simulink model "RefModel_RigInput"  (R2015b)
settings: configuration reference "CenterOutReachConfigSet" (kept outside this file)
undefined symbols (not defined in the file or in its folder): DiscIntNeverNeededParam, handAccelerationX, handAccelerationY, handAccelerationZ, HandSource, SimulinkParameter_TunableRigConfig
libraries: simulink x11, libBusSerialize x7, slrtlib x2, dspindex x1, libIntelSMI x1, xpcnilib x1, dspswit3 x1, commfilt2 x1
settings Model: Creator=djoshea  LastModifiedBy=shenoylab
settings ConfigSetRef: SourceLocation=Base Workspace

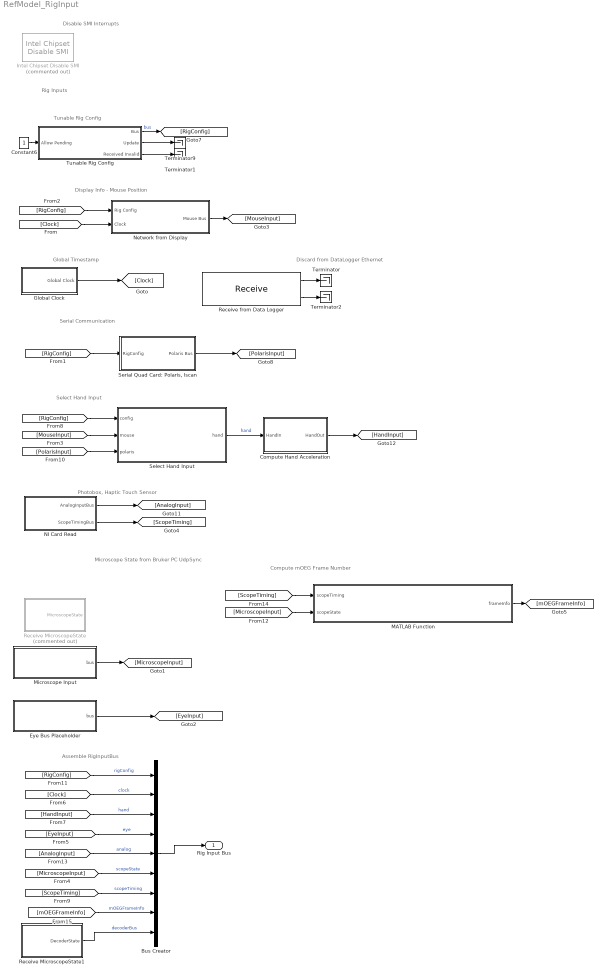
== system RefModel_RigInput ==
  note: Display Info - Mouse Position
  note: Serial Communication
  note: Global Timestamp
  note: Photobox, Haptic Touch Sensor
  note: Tunable Rig Config
  note: Select Hand Input
  note: Assemble RigInputBus
  note: Microscope State from Bruker PC UdpSync
  note: Disable SMI Interrupts
  note: Discard from DataLogger Ethernet
  note: Rig Inputs
  note: Compute mOEG Frame Number
  Bus Creator : BusCreator  Inputs=9  OutDataTypeStr=Bus: RigInputBus  NonVirtualBus=on
  Compute Hand Acceleration : Subsystem
  Constant6 : Constant  OutDataTypeStr=uint8
  Eye Bus Placeholder : MATLAB Function  AncestorBlock=libBusSerialize/Initialize Bus  TreatAsAtomicUnit=on  mask(Initialize Bus Block){busType=Bus: EyeInputBus}
      mask prompts: busType "Bus Type:"
      mask help: This block simply wraps an initializeBus_BusName() function and is useful for debugging where bus inputs are required. It acts essentially like a ground source for bus types.
      mask init:
      | BusSerialize.maskInitializeBusBlockUpdate(gcb);
  Global Clock : Subsystem
  Intel Chipset Disable SMI : libIntelSMI/Intel Chipset Disable SMI  Commented=on
  MATLAB Function : MATLAB Function  TreatAsAtomicUnit=on
  Microscope Input : MATLAB Function  AncestorBlock=libBusSerialize/Initialize Bus  TreatAsAtomicUnit=on  mask(Initialize Bus Block){busType=Bus: MicroscopeStateBus}
      mask prompts: busType "Bus Type:"
      mask help: This block simply wraps an initializeBus_BusName() function and is useful for debugging where bus inputs are required. It acts essentially like a ground source for bus types.
      mask init:
      | BusSerialize.maskInitializeBusBlockUpdate(gcb);
  NI Card Read : Subsystem
  Network from Display : Subsystem
  Receive MicroscopeState : Subsystem  Commented=on
  Receive MicroscopeState1 : Subsystem
  Receive from Data Logger : libBusSerialize/Receive   maskID=RigInfo.network.dataLoggerVLAN.ethernetId  sourceIP=RigInfo.network.dataLoggerVLAN.receiveFromIP  Receive2=RigInfo.network.dataLoggerVLAN.receiveAtPort  Receive3=1500  Receive4=0.001  udpID=0  ID=3
  Select Hand Input : MATLAB Function  TreatAsAtomicUnit=on
  "Serial Quad Card: Polaris, Iscan" : Subsystem
  Terminator{,1..2,9} (4 alike) : Terminator
  Tunable Rig Config : Subsystem  AncestorBlock=libBusSerialize/Serialized Bus Tunable Parameter  mask(BusSerialize Tunable Parameter Block){paramName='TunableRigConfig'}
      mask prompts: paramName "Parameter Name"
      mask help: This block provides the value of a tunable Simulink.Parameter into the model. Since tunable parameters with xPC target can only be doubles, the functions BusSerialize.createTunableParameter and BusSerialize.setTunableParameter automatically handle typecasting and update counter insertion, and this block handles update detection, typecasting, and reshaping back to the original form. Currently, variable size parameters are not supported.
      mask init:
      | BusSerialize.maskSerializedBusTunableParameterBlockUpdate(gcb);
      mask Display:
      | port_label('output', 1, paramName);
      | port_label('output', 2, 'Update');
      | port_label('output', 3, 'Received Invalid');
      | port_label('input', 1, 'Allow Pending');
  Rig Input Bus : Outport  OutDataTypeStr=Bus: RigInputBus  PortDimensions=1  BusOutputAsStruct=on
  wires:
  Global Clock/1(Global Clock) -> [Clock]
  Tunable Rig Config/2(Update) -> Terminator9/1
  Constant6/1 -> Tunable Rig Config/1(Allow Pending)
  [MouseInput] -> Select Hand Input/2(mouse)
  Network from Display/1(Mouse Bus) -> [MouseInput]
  [Clock] -> Bus Creator/2  "clock"
  [HandInput] -> Bus Creator/3  "hand"
  Tunable Rig Config/1(Bus) -> [RigConfig]  "bus"
  [RigConfig] -> Select Hand Input/1(config)
  "Serial Quad Card: Polaris, Iscan"/1(Polaris Bus) -> [PolarisInput]
  [PolarisInput] -> Select Hand Input/3(polaris)
  [AnalogInput] -> Bus Creator/5  "analog"
  Select Hand Input/1(hand) -> Compute Hand Acceleration/1(HandIn)  "hand"
  Bus Creator/1 -> Rig Input Bus/1
  Tunable Rig Config/3(Received Invalid) -> Terminator1/1
  Compute Hand Acceleration/1(HandOut) -> [HandInput]
  [RigConfig] -> "Serial Quad Card: Polaris, Iscan"/1(RigConfig)
  [Clock] -> Network from Display/2(Clock)
  [RigConfig] -> Network from Display/1(Rig Config)
  [MicroscopeInput] -> Bus Creator/6  "scopeState"
  Eye Bus Placeholder/1(bus) -> [EyeInput]
  [EyeInput] -> Bus Creator/4  "eye"
  Receive from Data Logger/1 -> Terminator/1
  Receive from Data Logger/2 -> Terminator2/1
  NI Card Read/1(AnalogInputBus) -> [AnalogInput]
  NI Card Read/2(ScopeTimingBus) -> [ScopeTiming]
  [ScopeTiming] -> Bus Creator/7  "scopeTiming"
  [RigConfig] -> Bus Creator/1  "rigConfig"
  MATLAB Function/1(frameInfo) -> [mOEGFrameInfo]
  [mOEGFrameInfo] -> Bus Creator/8  "mOEGFrameInfo"
  [ScopeTiming] -> MATLAB Function/1(scopeTiming)
  [MicroscopeInput] -> MATLAB Function/2(scopeState)
  Receive MicroscopeState1/1(DecoderState) -> Bus Creator/9  "decoderBus"
  Microscope Input/1(bus) -> [MicroscopeInput]

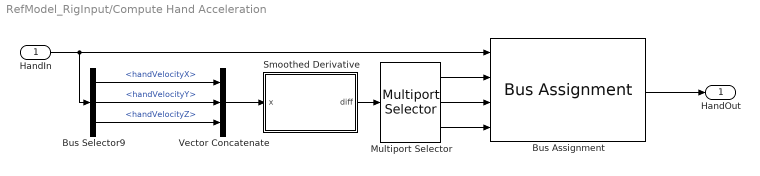
== system RefModel_RigInput/Compute Hand Acceleration ==
  HandIn : Inport  OutDataTypeStr=Bus: HandBus
  Bus Assignment : BusAssignment  AssignedSignals=handAccelerationX,handAccelerationY,handAccelerationZ
  Bus Selector9 : BusSelector  OutputSignals=handVelocityX,handVelocityY,handVelocityZ
  Multiport Selector : dspindex/Multiport Selector  rowsOrCols=Rows  idxCellArray={1,2,3}  idxErrMode=Clip Index
  Smoothed Derivative : Subsystem  mask{filterTau=0.05, Ts=0.001}
      mask prompts: filterTau "Smoothing Tau"; Ts "Sample Time"
  Vector Concatenate : Concatenate  NumInputs=3
  HandOut : Outport  OutDataTypeStr=Bus: HandBus
  wires:
  Bus Selector9/1 -> Vector Concatenate/1  "<handVelocityX>"
  Bus Selector9/2 -> Vector Concatenate/2  "<handVelocityY>"
  Bus Assignment/1 -> HandOut/1
  HandIn/1 -> Bus Selector9/1, Bus Assignment/1
  Bus Selector9/3 -> Vector Concatenate/3  "<handVelocityZ>"
  Vector Concatenate/1 -> Smoothed Derivative/1(x)
  Smoothed Derivative/1(diff) -> Multiport Selector/1
  Multiport Selector/1 -> Bus Assignment/2
  Multiport Selector/2 -> Bus Assignment/3
  Multiport Selector/3 -> Bus Assignment/4

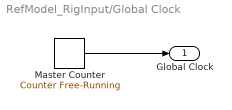
== system RefModel_RigInput/Global Clock ==
  Master Counter : simulink/Sources/Counter Free-Running  NumBits=32  tsamp=-1
  Global Clock : Outport  OutDataTypeStr=uint32  PortDimensions=1
  wires:
  Master Counter/1 -> Global Clock/1

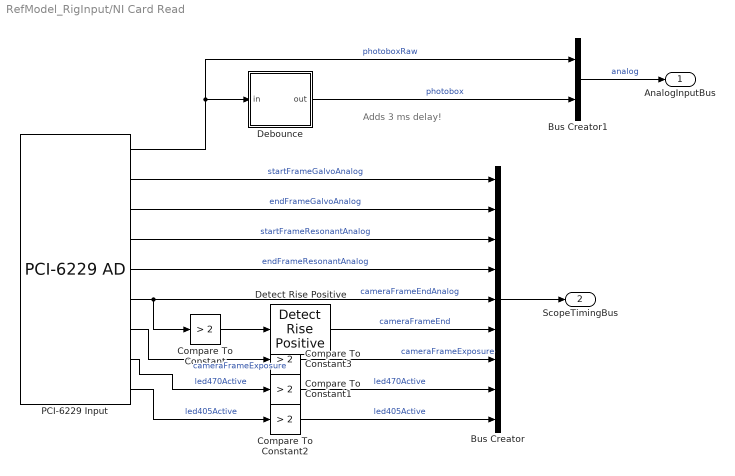
== system RefModel_RigInput/NI Card Read ==
  note: Adds 3 ms delay!
  Bus Creator : BusCreator  Inputs=9  OutDataTypeStr=Bus: ScopeTimingBus  NonVirtualBus=on
  Bus Creator1 : BusCreator  Inputs=2  OutDataTypeStr=Bus: AnalogInputBus  NonVirtualBus=on
  Compare To Constant{,1..3} (4 alike) : simulink/Logic and Bit Operations/Compare To Constant  relop=>  const=2  OutDataTypeStr=uint8
  Debounce : Stateflow chart  TreatAsAtomicUnit=on
  Detect Rise Positive : simulink/Logic and Bit Operations/Detect Rise Positive  vinit=0  InputProcessing=Inherited  OutDataTypeStr=uint8
  PCI-6229 Input : xpcnilib/A//D/M Series/PCI-6229 AD  channel=[1 2 3 4 5 6 7 8 9]  range=[10]  coupling=[0]  scantime=5e-6  sampletime=-1  slot=-1
  AnalogInputBus : Outport  OutDataTypeStr=Bus: AnalogInputBus
  ScopeTimingBus : Outport  Port=2  OutDataTypeStr=Bus: ScopeTimingBus  PortDimensions=1
  wires:
  PCI-6229 Input/4 -> Bus Creator/3  "startFrameResonantAnalog"
  PCI-6229 Input/5 -> Bus Creator/4  "endFrameResonantAnalog"
  PCI-6229 Input/3 -> Bus Creator/2  "endFrameGalvoAnalog"
  PCI-6229 Input/2 -> Bus Creator/1  "startFrameGalvoAnalog"
  Bus Creator/1 -> ScopeTimingBus/1
  PCI-6229 Input/1 -> Debounce/1(in), Bus Creator1/1  "photoboxRaw"
  Debounce/1(out) -> Bus Creator1/2  "photobox"
  Bus Creator1/1 -> AnalogInputBus/1  "analog"
  PCI-6229 Input/6 -> Compare To Constant/1, Bus Creator/5  "cameraFrameEndAnalog"
  Compare To Constant/1 -> Detect Rise Positive/1
  Detect Rise Positive/1 -> Bus Creator/6  "cameraFrameEnd"
  PCI-6229 Input/8 -> Compare To Constant1/1  "led470Active"
  PCI-6229 Input/7 -> Compare To Constant3/1  "cameraFrameExposure"
  PCI-6229 Input/9 -> Compare To Constant2/1  "led405Active"
  Compare To Constant1/1 -> Bus Creator/8  "led470Active"
  Compare To Constant2/1 -> Bus Creator/9  "led405Active"
  Compare To Constant3/1 -> Bus Creator/7  "cameraFrameExposure"

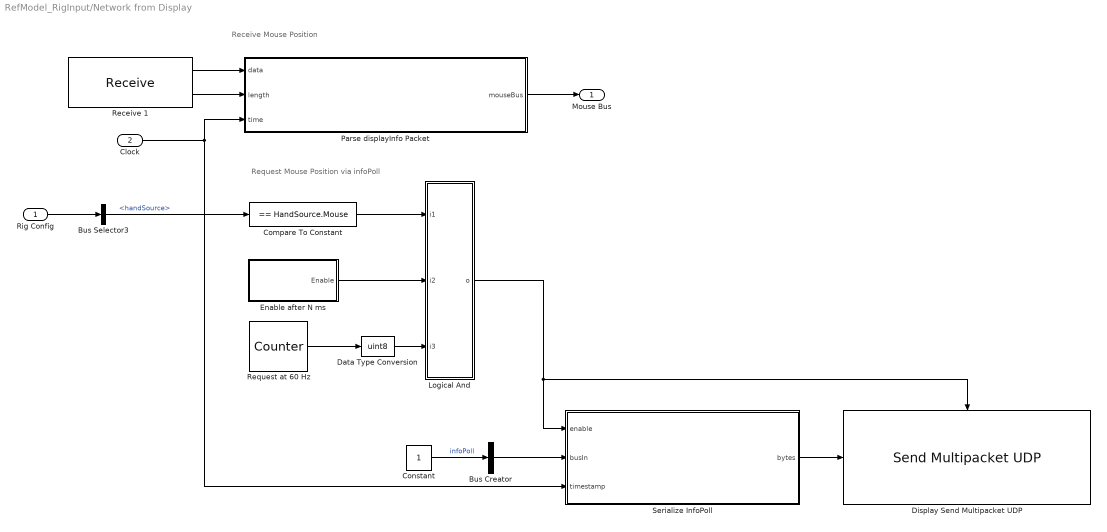
== system RefModel_RigInput/Network from Display ==
  note: Request Mouse Position via infoPoll
  note: Receive Mouse Position
  Rig Config : Inport  OutDataTypeStr=Bus: RigConfigBus
  Clock : Inport  Port=2  PortDimensions=1
  Bus Creator : BusCreator  Inputs=1  OutDataTypeStr=Bus: DisplayInfoRequestBus  NonVirtualBus=on
  Bus Selector3 : BusSelector  OutputSignals=handSource
  Compare To Constant : simulink/Logic and Bit Operations/Compare To Constant  relop===  const=HandSource.Mouse  OutDataTypeStr=uint8
  Constant : Constant  OutDataTypeStr=uint8
  Data Type Conversion : DataTypeConversion  OutDataTypeStr=uint8
  Display Send Multipacket UDP : libBusSerialize/Send Multipacket UDP  transmitId=11  sourceIP=RigInfo.network.displayVLAN.sourceIP  sourcePort=RigInfo.network.displayVLAN.sourcePort  destIP=RigInfo.network.displayVLAN.broadcastIP  destPort=RigInfo.network.displayVLAN.destPort  destMac=RigInfo.network.displayVLAN.broadcastMac  deviceID=RigInfo.network.displayVLAN.ethernetId  prependHeader=on
  Enable after N ms : Subsystem  mask{const=100}
      mask prompts: const "Initial Wait Ticks"
      mask TypeOptions const:
      | Compare
      | To Constant/const
  Logical And : MATLAB Function  TreatAsAtomicUnit=on
  Parse displayInfo Packet : MATLAB Function  TreatAsAtomicUnit=on
  Receive 1 : libBusSerialize/Receive   maskID=RigInfo.network.displayVLAN.ethernetId  sourceIP=RigInfo.network.displayVLAN.receiveFromIP  Receive2=RigInfo.network.displayVLAN.receiveAtPort  Receive3=1500  Receive4=0.001  udpID=0  ID=5
  Request at 60 Hz : dspswit3/Counter  Direction=Up  CountEvent=Free running  CounterSize=User defined  MaxCount=16  InitialCount=0  Output=Hit  HitValue=5  ResetInput=off  SamplesPerFrame=1  Ts=0.001  CntDtype=double  HitDtype=Logical
  Serialize InfoPoll : MATLAB Function  AncestorBlock=libBusSerialize/fn2  TreatAsAtomicUnit=on  mask(BusSerialize: serialize block){busType=Bus: DisplayInfoRequestBus, groupType=Parameter, groupName='infoPoll'}
      mask prompts: busType "Bus Type"; groupType "Group Type"; groupName "Group Name"
      mask help: Select the bus type below to serialize.
      mask init:
      | BusSerialize.maskSerializeWithDataLoggerHeaderBlockUpdate(gcb)
  Mouse Bus : Outport  OutDataTypeStr=Bus: MouseInputBus  PortDimensions=1
  wires:
  Parse displayInfo Packet/1(mouseBus) -> Mouse Bus/1
  Receive 1/1 -> Parse displayInfo Packet/1(data)
  Receive 1/2 -> Parse displayInfo Packet/2(length)
  Bus Selector3/1 -> Compare To Constant/1  "<handSource>"
  Rig Config/1 -> Bus Selector3/1
  Constant/1 -> Bus Creator/1  "infoPoll"
  Clock/1 -> Serialize InfoPoll/3(timestamp), Parse displayInfo Packet/3(time)
  Bus Creator/1 -> Serialize InfoPoll/2(busIn)
  Serialize InfoPoll/1(bytes) -> Display Send Multipacket UDP/1
  Request at 60 Hz/1 -> Data Type Conversion/1
  Logical And/1(o) -> Display Send Multipacket UDP/Enable, Serialize InfoPoll/1(enable)
  Enable after N ms/1(Enable) -> Logical And/2(i2)
  Compare To Constant/1 -> Logical And/1(i1)
  Data Type Conversion/1 -> Logical And/3(i3)

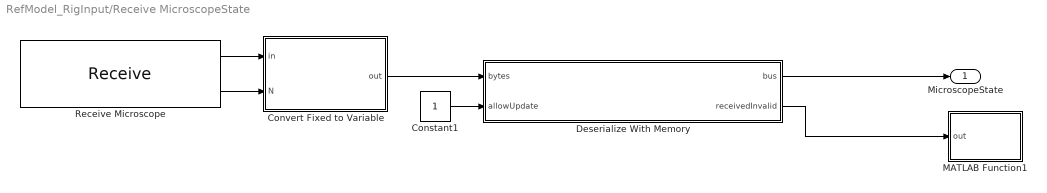
== system RefModel_RigInput/Receive MicroscopeState ==
  Constant1 : Constant  OutDataTypeStr=uint8
  Convert Fixed to Variable : MATLAB Function  TreatAsAtomicUnit=on  mask(Converts Variable-size to fixed-size array){bufferSize=1500}
      mask prompts: bufferSize "Buffer Size"
      mask help: Specify maximum input size.
  Deserialize With Memory : MATLAB Function  AncestorBlock=libBusSerialize/Deserialize With Memory  TreatAsAtomicUnit=on  mask(Deserialize Bus With Internal Memory){busType=Bus: MicroscopeStateBus}
      mask prompts: busType "Bus Type:"
      mask help:
      | This block deserializes a uint8 bytestream into a specific bus type. When the input changes, the block will deserialize the new input, and the deserialization is successful, it will internally store the updated bus.
      |
      | If allowUpdate is high at that point, the new bus value will be output immediately and update will be driven high. If not, pendingUpdate will be driven high, and the updated bus will be held in an internal persistent variable. When allowUpdate goes high, this updated bus will be passed to the output, and update will be driven high.
      |
      | If an invalid serialized bus is received, receivedInvalid will be driven high, and the bus output will not change from its previously stored value. If the initial value sent to this block is invalid, a default initialized bus will be output with all zeros or empty bus elements.
      mask init:
      | BusSerialize.maskDeserializeMemoryBlockUpdate(gcb);
  MATLAB Function1 : MATLAB Function  TreatAsAtomicUnit=on
  Receive Microscope : libBusSerialize/Receive   maskID=RigInfo.network.scopeVLAN.ethernetId  sourceIP=RigInfo.network.scopeVLAN.receiveFromIP  Receive2=RigInfo.network.scopeVLAN.receiveAtPort  Receive3=1500  Receive4=0.001  udpID=0  ID=2
  MicroscopeState : Outport  OutDataTypeStr=Bus: MicroscopeStateBus
  wires:
  Receive Microscope/1 -> Convert Fixed to Variable/1(in)
  Convert Fixed to Variable/1(out) -> Deserialize With Memory/1(bytes)
  Constant1/1 -> Deserialize With Memory/2(allowUpdate)
  Deserialize With Memory/1(bus) -> MicroscopeState/1
  Deserialize With Memory/2(receivedInvalid) -> MATLAB Function1/1(out)
  Receive Microscope/2 -> Convert Fixed to Variable/2(N)

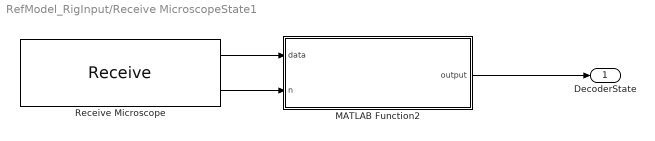
== system RefModel_RigInput/Receive MicroscopeState1 ==
  MATLAB Function2 : MATLAB Function  TreatAsAtomicUnit=on
  Receive Microscope : libBusSerialize/Receive   maskID=RigInfo.network.scopeVLAN.ethernetId  sourceIP=RigInfo.network.scopeVLAN.receiveFromIP  Receive2=RigInfo.network.scopeVLAN.receiveAtPort  Receive3=1500  Receive4=0.001  udpID=0  ID=2
  DecoderState : Outport  OutDataTypeStr=Bus: DecoderBus
  wires:
  Receive Microscope/1 -> MATLAB Function2/1(data)
  Receive Microscope/2 -> MATLAB Function2/2(n)
  MATLAB Function2/1(output) -> DecoderState/1

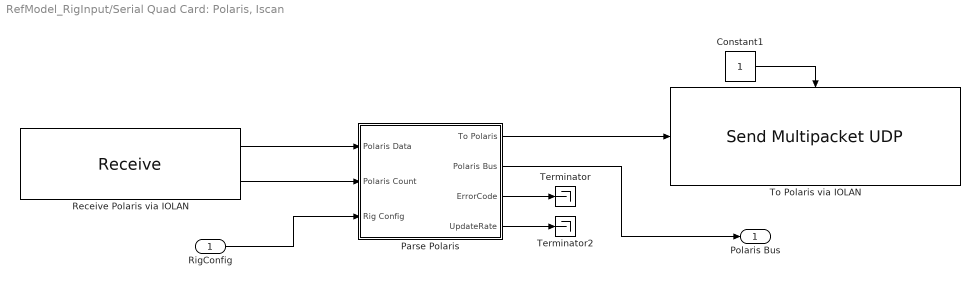
== system RefModel_RigInput/Serial Quad Card: Polaris, Iscan ==
  RigConfig : Inport
  Constant1 : Constant
  Parse Polaris : Subsystem
  Receive Polaris via IOLAN : libBusSerialize/Receive   maskID=RigInfo.network.serialVLAN.ethernetId  sourceIP=RigInfo.network.serialVLAN.receiveFromIP  Receive2=RigInfo.network.serialVLAN.receiveAtPort  Receive3=1024  Receive4=0.001  udpID=0  ID=7
  Terminator : Terminator
  Terminator2 : Terminator
  To Polaris via IOLAN : libBusSerialize/Send Multipacket UDP  transmitId=1  sourceIP=RigInfo.network.serialVLAN.sourceIP  sourcePort=RigInfo.network.serialVLAN.sourcePort  destIP=RigInfo.network.serialVLAN.broadcastIP  destPort=RigInfo.network.serialVLAN.destPort  destMac=RigInfo.network.serialVLAN.broadcastMac  deviceID=RigInfo.network.serialVLAN.ethernetId  prependHeader=off
  Polaris Bus : Outport
  wires:
  Receive Polaris via IOLAN/1 -> Parse Polaris/1(Polaris Data)
  Receive Polaris via IOLAN/2 -> Parse Polaris/2(Polaris Count)
  Constant1/1 -> To Polaris via IOLAN/Enable
  Parse Polaris/1(To Polaris) -> To Polaris via IOLAN/1
  Parse Polaris/3(ErrorCode) -> Terminator/1
  RigConfig/1 -> Parse Polaris/3(Rig Config)
  Parse Polaris/4(UpdateRate) -> Terminator2/1
  Parse Polaris/2(Polaris Bus) -> Polaris Bus/1

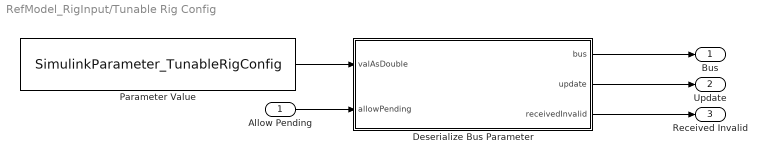
== system RefModel_RigInput/Tunable Rig Config ==
  Allow Pending : Inport
  Deserialize Bus Parameter : MATLAB Function  TreatAsAtomicUnit=on
  Parameter Value : Constant  Value=SimulinkParameter_TunableRigConfig  OutDataTypeStr=double
  Bus : Outport  PortDimensions=1
  Update : Outport  Port=2  OutDataTypeStr=uint8  PortDimensions=1
  Received Invalid : Outport  Port=3  OutDataTypeStr=uint8  PortDimensions=1
  wires:
  Parameter Value/1 -> Deserialize Bus Parameter/1(valAsDouble)
  Allow Pending/1 -> Deserialize Bus Parameter/2(allowPending)
  Deserialize Bus Parameter/3(receivedInvalid) -> Received Invalid/1
  Deserialize Bus Parameter/1(bus) -> Bus/1
  Deserialize Bus Parameter/2(update) -> Update/1

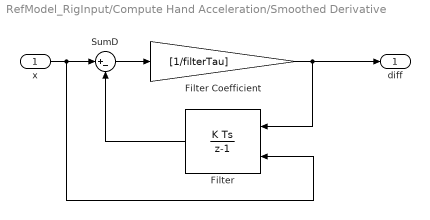
== system RefModel_RigInput/Compute Hand Acceleration/Smoothed Derivative ==
  x : Inport
  Filter : DiscreteIntegrator  DisableCoverage=on  gainval=[1.0 1.0 1.0]  InitialConditionSource=external  InitialConditionSetting=State (most efficient)  SampleTime=Ts  OutDataTypeStr=double  ICPrevOutput=DiscIntNeverNeededParam  ICPrevScaledInput=DiscIntNeverNeededParam
  Filter Coefficient : Gain  Gain=[1/filterTau]  OutDataTypeStr=double  SampleTime=Ts
  SumD : Sum  DisableCoverage=on  Inputs=|+-  OutDataTypeStr=double  SampleTime=Ts
  diff : Outport  PortDimensions=3
  wires:
  x/1 -> SumD/1, Filter/2
  Filter/1 -> SumD/2
  SumD/1 -> Filter Coefficient/1
  Filter Coefficient/1 -> Filter/1, diff/1

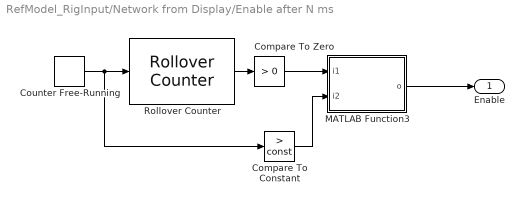
== system RefModel_RigInput/Network from Display/Enable after N ms ==
  Compare To Constant : simulink/Logic and Bit Operations/Compare To Constant  relop=>  const=const  OutDataTypeStr=uint8
  Compare To Zero : simulink/Logic and Bit Operations/Compare To Zero  relop=>  OutDataTypeStr=uint8
  Counter Free-Running : simulink/Sources/Counter Free-Running  NumBits=16  tsamp=-1
  MATLAB Function3 : MATLAB Function  TreatAsAtomicUnit=on
  Rollover Counter : slrtlib/Incremental Encoder/Utilities/Rollover/Rollover Counter   InitialValue=0  RolloverThreshold=2^15
  Enable : Outport
  wires:
  MATLAB Function3/1(o) -> Enable/1
  Compare To Constant/1 -> MATLAB Function3/2(i2)
  Compare To Zero/1 -> MATLAB Function3/1(i1)
  Rollover Counter/1 -> Compare To Zero/1
  Counter Free-Running/1 -> Compare To Constant/1, Rollover Counter/1

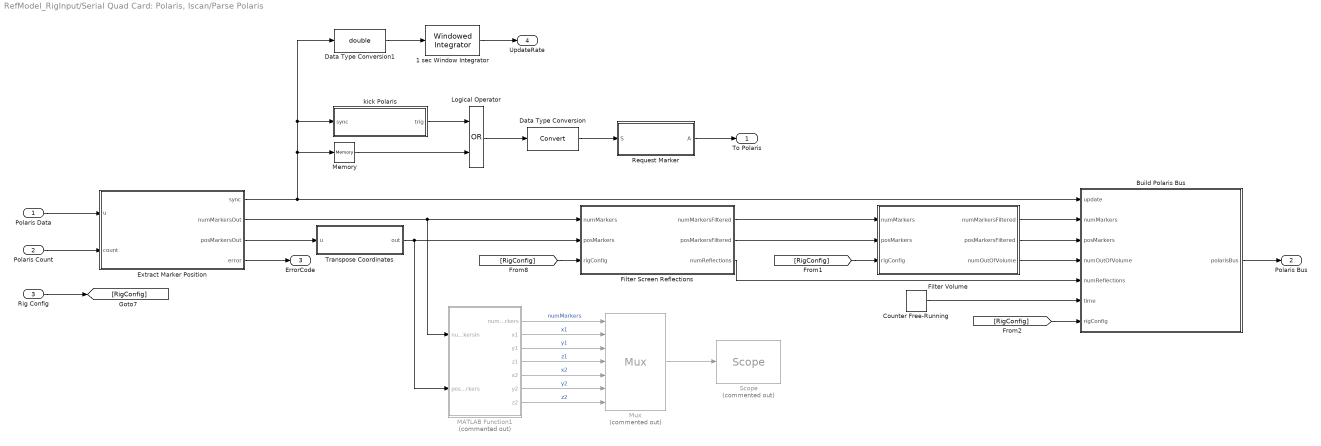
== system RefModel_RigInput/Serial Quad Card: Polaris, Iscan/Parse Polaris ==
  Polaris Data : Inport  OutDataTypeStr=uint8
  Polaris Count : Inport  Port=2
  Rig Config : Inport  Port=3  OutDataTypeStr=Bus: RigConfigBus
  1 sec Window Integrator : commfilt2/Windowed Integrator  integperiod=1000  roundingMode=Floor  overflowMode=off  InputProcessing=Columns as channels (frame based)
  Build Polaris Bus : MATLAB Function  TreatAsAtomicUnit=on
  Counter Free-Running : simulink/Sources/Counter Free-Running  NumBits=32  tsamp=0.001
  Data Type Conversion : DataTypeConversion
  Data Type Conversion1 : DataTypeConversion  OutDataTypeStr=double
  Extract Marker Position : MATLAB Function  TreatAsAtomicUnit=on
  Filter Screen Reflections : MATLAB Function  TreatAsAtomicUnit=on
  Filter Volume : MATLAB Function  TreatAsAtomicUnit=on
  Logical Operator : Logic  Operator=OR  AllPortsSameDT=off  OutDataTypeStr=boolean
  MATLAB Function1 : MATLAB Function  Commented=on  TreatAsAtomicUnit=on
  Memory : Memory  InheritSampleTime=on
  Mux : Mux  Commented=on  Inputs=7
      settings: DisplayOption=signals
  Request Marker : MATLAB Function  TreatAsAtomicUnit=on
  "Scope " : slrtlib/Displays and Logging/Scope   Commented=on  scopeno=1  scopetype=Target  autostart=on  viewmode=Numerical  formatstr='%15.6f'  grid=on  ylimits=[0,0]  nosamples=250  noprepostsamples=0  interleave=1  triggermode=FreeRun  triggersignal=1  trigsignalfromport=off  triggerlevel=0.0  triggerslope=Either  triggerscope=1  triggersample=0  filename=data.dat  mode=Lazy  writesize=512  autorestart=off  dynamicfilemode=off  maxwritefilesize=512*1024^2
  Transpose Coordinates : MATLAB Function  TreatAsAtomicUnit=on
  kick Polaris : MATLAB Function  TreatAsAtomicUnit=on
  To Polaris : Outport  OutDataTypeStr=uint8
  Polaris Bus : Outport  Port=2  OutDataTypeStr=Bus: PolarisInputBus
  ErrorCode : Outport  Port=3
  UpdateRate : Outport  Port=4
  wires:
  1 sec Window Integrator/1 -> UpdateRate/1
  Data Type Conversion1/1 -> 1 sec Window Integrator/1
  Memory/1 -> Logical Operator/2
  Extract Marker Position/4(error) -> ErrorCode/1
  Transpose Coordinates/1(out) -> MATLAB Function1/2(posMarkers), Filter Screen Reflections/2(posMarkers)
  kick Polaris/1(trig) -> Logical Operator/1
  Logical Operator/1 -> Data Type Conversion/1
  Request Marker/1(A) -> To Polaris/1
  Extract Marker Position/3(posMarkersOut) -> Transpose Coordinates/1(u)
  Extract Marker Position/2(numMarkersOut) -> MATLAB Function1/1(numMarkersIn), Filter Screen Reflections/1(numMarkers)
  Polaris Data/1 -> Extract Marker Position/1(u)
  Polaris Count/1 -> Extract Marker Position/2(count)
  [RigConfig] -> Filter Screen Reflections/3(rigConfig)
  MATLAB Function1/1(numMarkers) -> Mux/1  "numMarkers"
  MATLAB Function1/2(x1) -> Mux/2  "x1"
  MATLAB Function1/3(y1) -> Mux/3  "y1"
  MATLAB Function1/4(z1) -> Mux/4  "z1"
  MATLAB Function1/5(x2) -> Mux/5  "x2"
  MATLAB Function1/6(y2) -> Mux/6  "y2"
  MATLAB Function1/7(z2) -> Mux/7  "z2"
  Mux/1 -> "Scope "/1
  Extract Marker Position/1(sync) -> Memory/1, Data Type Conversion1/1, kick Polaris/1(sync), Build Polaris Bus/1(update)
  Data Type Conversion/1 -> Request Marker/1(S)
  Filter Screen Reflections/1(numMarkersFiltered) -> Filter Volume/1(numMarkers)
  Filter Screen Reflections/2(posMarkersFiltered) -> Filter Volume/2(posMarkers)
  Filter Volume/1(numMarkersFiltered) -> Build Polaris Bus/2(numMarkers)
  Filter Volume/2(posMarkersFiltered) -> Build Polaris Bus/3(posMarkers)
  Filter Screen Reflections/3(numReflections) -> Build Polaris Bus/5(numReflections)
  Filter Volume/3(numOutOfVolume) -> Build Polaris Bus/4(numOutOfVolume)
  Rig Config/1 -> [RigConfig]
  [RigConfig] -> Filter Volume/3(rigConfig)
  [RigConfig] -> Build Polaris Bus/7(rigConfig)
  Build Polaris Bus/1(polarisBus) -> Polaris Bus/1
  Counter Free-Running/1 -> Build Polaris Bus/6(time)

== matlab function RefModel_RigInput/Network from Display/Serialize InfoPoll ==
  data: enable input uint8 size=1; busIn input Bus: DisplayInfoRequestBus size=1; bytes output uint8 size=45; timestamp input uint32 size=1
function bytes = dataLoggerSerialize(enable, busIn, timestamp)
%#codegen
    if enable
        bytes = serializeBusWithDataLoggerHeader_DisplayInfoRequestBus(busIn, uint8(BusSerialize.GroupTypes.Parameter), uint8('infoPoll'), timestamp);
    else
        bytes = zeros(0, 1, 'uint8');
    end
end

== matlab function RefModel_RigInput/Network from Display/Parse displayInfo Packet ==
  data: data input; length input; mouseBus output Bus: MouseInputBus size=1; time input uint32 size=1
function mouseBus  = parseUDPFromDisplayPC(data, length, time)
%#codegen

persistent pMouse;
if isempty(pMouse)
    pMouse = initializeBus_MouseInputBus();
end
mouseBus = pMouse;
update = uint8(0);
screenFlip = uint8(0);

header = uint8('<displayInfo>')';
headerLength = numel(header);

nBytes = uint16(1 + 8 + 8 + 1 + headerLength);
offset = uint16(1);

if(length < nBytes)
    return;
end

if any(header(1:headerLength) ~= data(1:headerLength))
    return;
end
offset = offset + uint16(headerLength);

%screenFlip = uint8(data(offset));
offset = offset + 1;

mouseBus.mouseX = typecast(data(offset:offset+7), 'double');
offset = offset + 8;

mouseBus.mouseY = typecast(data(offset:offset+7), 'double');
offset = offset + 8;

mouseBus.mouseClick = uint8(data(offset));
%offset = offset + 1;

mouseBus.update = uint8(1);

% compute simple non-uniformly sampled derivatives
persistent pX;
persistent pY;
persistent pTime;
if mouseBus.update
    if isempty(pX) || isempty(pY)
        pX = mouseBus.mouseX;
        pY = mouseBus.mouseY;
    end
    if isempty(pTime)
        pTime = time;
    end
    
    if double(time - pTime) > 0
        mouseBus.mouseVelX = (double(mouseBus.mouseX) - double(pX)) / double(time - pTime);
        mouseBus.mouseVelY = (double(mouseBus.mouseY) - double(pY)) / double(time - pTime);
    end
    
    pX = mouseBus.mouseX;
    pY = mouseBus.mouseY;
    pTime = time;
end

== matlab function RefModel_RigInput/Serial Quad Card: Polaris, Iscan/Parse Polaris/Build Polaris Bus ==
  data: update input; numMarkers input; polarisBus output Bus: PolarisInputBus size=1; posMarkers input; numOutOfVolume input; numReflections input; time input uint32 size=1; rigConfig input
function polarisBus = buildPolarisBus(update, numMarkers, posMarkers, numOutOfVolume, numReflections, time, rigConfig)

polarisBus = initializeBus_PolarisInputBus();
polarisBus.update = uint8(update);
if numMarkers == uint8(1)
    polarisBus.markerSeen = uint8(1);
    polarisBus.markerX = posMarkers(1, 1);
    polarisBus.markerY = posMarkers(1, 2);
    polarisBus.markerZ = posMarkers(1, 3);
    
    if polarisBus.markerZ < rigConfig.polarisThreshTouchingZ
        polarisBus.touchingScreen = uint8(1);
    end
end

polarisBus.numMakersInVolume = uint8(numMarkers);
polarisBus.numReflections = uint8(numReflections);
polarisBus.numMarkersOutOfVolume = uint8(numOutOfVolume);

% compute simple non-uniformly sampled derivatives
persistent pX;
persistent pY;
persistent pZ;
persistent pVelX;
persistent pVelY;
persistent pVelZ;
persistent pTime;

if isempty(pVelX) || isempty(pVelY) || isempty(pVelZ)
    pVelX = 0;
    pVelY = 0;
    pVelZ = 0;
end

if polarisBus.update
    if isempty(pX) || isempty(pY) || isempty(pZ)       
        pX = polarisBus.markerX;
        pY = polarisBus.markerY;
        pZ = polarisBus.markerZ;
    end  
    
    if polarisBus.markerSeen % update velocities with simple first order difference
        if isempty(pTime)
            pTime = time;
        end

        if double(time - pTime) > 0
            pVelX = (double(polarisBus.markerX) - double(pX)) / double(time - pTime) * 1000;
            pVelY = (double(polarisBus.markerY) - double(pY)) / double(time - pTime) * 1000;
            pVelZ = (double(polarisBus.markerZ) - double(pZ)) / double(time - pTime) * 1000;    
        end
    end
     
    pX = polarisBus.markerX;
    pY = polarisBus.markerY;
    pZ = polarisBus.markerZ;
    pTime = time;
end

polarisBus.markerVelX = pVelX;
polarisBus.markerVelY = pVelY;
polarisBus.markerVelZ = pVelZ;

end

== matlab function RefModel_RigInput/Serial Quad Card: Polaris, Iscan/Parse Polaris/MATLAB Function1 ==
  data: numMarkersIn input; numMarkers output; posMarkers input; x1 output; y1 output; z1 output; x2 output; y2 output; z2 output
function [numMarkers, x1, y1, z1, x2, y2, z2] = extractRaw(numMarkersIn, posMarkers)

numMarkers = double(numMarkersIn);
x1 = posMarkers(1, 1);
y1 = posMarkers(1, 2);
z1 = posMarkers(1, 3);
x2 = posMarkers(2, 1);
y2 = posMarkers(2, 2);
z2 = posMarkers(2, 3);

end

== matlab function RefModel_RigInput/Receive MicroscopeState/MATLAB Function1 ==
  data: out input uint8
function print(out)
%#codegen

if out > 0
    coder.ceval('printf', ['Error: Received invalid bus!' uint8([10 0])]);
end

== matlab function RefModel_RigInput/MATLAB Function ==
  data: scopeTiming input Bus: ScopeTimingBus size=1; scopeState input Bus: MicroscopeStateBus size=1; frameInfo output Bus: mOEGFrameInfoBus size=1
function frameInfo = buildmOEGFrameInfo(scopeTiming, scopeState)
%#codegen

persistent pFrameCount;
persistent pFileCount;
persistent pLastFileFrameCount;
persistent pIsAcquiring;

if isempty(pFrameCount) || isempty(pFileCount) || isempty(pLastFileFrameCount) || isempty(pIsAcquiring)
    pFileCount = uint32(0);
    pFrameCount = uint32(0);
    pLastFileFrameCount = uint32(0); 
    pIsAcquiring = uint8(0);
end

% reset frame count if file counter changes (or on startup)
if pFileCount ~= scopeState.cameraFileCounter
    pFileCount = uint32(scopeState.cameraFileCounter);
    
    if pFrameCount > 0
        pLastFileFrameCount = pFrameCount - 1; % would be on the nth + 1 frame  
    end
    pFrameCount = uint32(0);
    
elseif pIsAcquiring && ~scopeState.cameraIsAcquiring
    % we just finished a file, cache the frame count
    if pFrameCount > 0 % check that we didn't reset already
        pLastFileFrameCount = pFrameCount - 1; % would be on the nth + 1 frame
    end
    pFrameCount = uint32(0);
end

% increment frame count if frameEnd and we're acquiring
if scopeTiming.cameraFrameEnd && scopeState.cameraIsAcquiring
    pFrameCount = pFrameCount + uint32(1);
end

pIsAcquiring = uint8(scopeState.cameraIsAcquiring);

frameInfo = initializeBus_mOEGFrameInfoBus();
frameInfo.mOEGIsAcquiring = uint8(scopeState.cameraIsAcquiring);
frameInfo.mOEGFileNumber = pFileCount;
frameInfo.mOEGFrameNumber = pFrameCount;
frameInfo.mOEGLastFileFrameCount = pLastFileFrameCount;

end

== matlab function RefModel_RigInput/Receive MicroscopeState1/MATLAB Function2 ==
  data: data input uint8; output output Bus: DecoderBus; n input
function output = parseBrukerDecodePacket(data, n)
%#codegen
NUM_CONDITIONS = 4;

output = initializeBus_DecoderBus();

if ( n > 4 && (data(1) == uint8('#')) && (data(2) == uint8('U')) )
    output.decoderUpdate = uint8(1);
    output.decodeConditionId = typecast(data(3:4), 'uint16');
    
    offset = 5;
    for ii = 1:NUM_CONDITIONS    
        output.conditionPredictionLikelihood(ii) = typecast(data(offset : offset+7), 'double');
        offset = offset + 8;
    end
    
    endInd = min(300, n);
    output.classifierInfo = data(offset:endInd);
    
else
    output.decodeConditionId = uint16(0);
    output.conditionPredictionLikelihood = double(zeros(4,1));
    output.classifierInfo = zeros([0 1], 'uint8');
    
end

== stateflow chart RefModel_RigInput/NI Card Read/Debounce ==
  state WaitOn
    entry: out = uint8(0);
  state Off
    entry: out = uint8(0);
  state WaitOff
    entry: out = uint8(1);
  state On
    entry: out = uint8(1);
  (default) -> Off
  Off -> WaitOn : [in>threshHigh]
  WaitOn -> On [order 2] : after(nWait, tick)
  WaitOn -> Off [order 1] : [in <= threshHigh]
  WaitOff -> Off [order 2] : after(nWait, tick)
  WaitOff -> On [order 1] : [in >= threshLow]
  On -> WaitOff : [in < threshLow]
  data: in input double size=1; out output uint8 size=1; threshLow constant double size=1 =1.0; threshHigh constant double size=1 =1.5; nWait constant uint16 size=1 =3

== matlab function RefModel_RigInput/Microscope Input ==
  data: bus output Bus: MicroscopeStateBus size=1
function bus = initialize_MicroscopeStateBus()
%#codegen 

    bus = initializeBus_MicroscopeStateBus();

end

== matlab function RefModel_RigInput/Receive MicroscopeState/Deserialize With Memory ==
  data: bytes input; bus output Bus: MicroscopeStateBus size=1; allowUpdate input uint8 size=1; receivedInvalid output uint8 size=1
function [bus, receivedInvalid] = deserializeWithMemory(bytes, allowUpdate)
%#codegen

    % external cached output
    persistent pBusOut;
    if isempty(pBusOut)
        pBusOut = initializeBus_MicroscopeStateBus();
    end

    receivedInvalid = uint8(1);

    receivedInvalid = uint8(0);
    if allowUpdate && ~isempty(bytes)
        [bus, valid] = deserializeBus_MicroscopeStateBus(bytes);
        if valid
            % update internal cache
            pBusOut = bus;
        else
            % don't update internal cache, output internal cache
            bus = pBusOut;
            receivedInvalid = uint8(1);
        end
    else
        bus = pBusOut;
    end
end

== matlab function RefModel_RigInput/Select Hand Input ==
  data: config input Bus: RigConfigBus size=1; hand output Bus: HandBus size=1; mouse input Bus: MouseInputBus size=1; polaris input Bus: PolarisInputBus size=1
function hand = selectHandInput(config, mouse, polaris)
%#codegen

% initialize first so that we don't need to worry about assignment order
hand = initializeBus_HandBus();

hand.handSource = config.handSource;

switch config.handSource
    case HandSource.Mouse
        hand.handUpdate = mouse.update;
        hand.handSeen = uint8(1); % mouse always seen
        hand.handOnDevice = uint8(1); % mouse always "on device"
        
        hand.handX = mouse.mouseX;
        hand.handY = mouse.mouseY; 
        
        % let click sets handZ = 0, and indicates touching screen
        if mouse.mouseClick
            hand.handZ = 0;
            hand.handTouching = uint8(1);
        else
            hand.handZ = 100;
            hand.handTouching = uint8(0);
        end
        
        hand.handVelocityX = mouse.mouseVelX;
        hand.handVelocityY = mouse.mouseVelY;
        hand.handVelocityZ = 0;
        
    case HandSource.Polaris
        hand.handUpdate = polaris.update;
        hand.handSeen = polaris.markerSeen;
        hand.handTouching = polaris.touchingScreen;
        hand.handX = polaris.markerX;
        hand.handY = polaris.markerY;
        hand.handZ = polaris.markerZ;
        
        hand.handVelocityX = polaris.markerVelX;
        hand.handVelocityY = polaris.markerVelY;
        hand.handVelocityZ = polaris.markerVelZ;   
end

hand.handSpeed = sqrt(hand.handVelocityX.^2 + hand.handVelocityY.^2 + hand.handVelocityZ.^2);
hand.handMoving = uint8(hand.handSpeed > config.moveSpeedThresh);

== matlab function RefModel_RigInput/Serial Quad Card: Polaris, Iscan/Parse Polaris/Filter Screen Reflections ==
  data: numMarkers input; numMarkersFiltered output; posMarkers input; rigConfig input; posMarkersFiltered output; numReflections output
function [numMarkersFiltered,posMarkersFiltered,numReflections] = filterScreenReflections(...
    numMarkers, posMarkers, rigConfig)

% from rigConfig parameter:
% distThresh : maximum distance in x,y and from screen for pairs of markers
%   to be considered reflections
% screenZ : the coordinates of the screen plane in Z
% signAwayFromScreen : if 1, the reflection will have a lower Z value than
%   the actual marker, if -1, the reflection will have a higher Z value than
%   the actual marker.
distThreshXY = rigConfig.polarisReflectionDistanceThreshXY;
screenZ = rigConfig.polarisOrigin(3);
distThreshZ = rigConfig.polarisReflectionDistanceThreshZ;

numReflections = uint8(0);

if numMarkers < 2
    % cannot have any reflections
    posMarkersFiltered = posMarkers;
    numMarkersFiltered = numMarkers;
    return;
else
    posMarkersFiltered = 0 * posMarkers;
    numMarkersFiltered = uint8(0);
end

idxX = uint8(1);
idxY = uint8(2);
idxZ = uint8(3);

% we're looking for pairs of markers that have similar values in x, y and
% values of z located near screenZ

foundReflection = zeros(1, size(posMarkers,1), 'uint8');
remove = zeros(1, size(posMarkers, 1), 'uint8');

% loop over markers
for i = 1:numMarkers
    if remove(i) || foundReflection(i)
        continue;
    end
    
    % loop over other markers
    for j = i+1:numMarkers
        if remove(j) || foundReflection(i)
            continue;
        end
        
        % if i & j are close to each other in x,y and close to the screen in z
        if abs(posMarkers(i, idxX) - posMarkers(j, idxX)) <= distThreshXY && ...
           abs(posMarkers(i, idxY) - posMarkers(j, idxY)) <= distThreshXY && ...
           abs(posMarkers(i, idxZ) - screenZ) <= distThreshZ && ...
           abs(posMarkers(j, idxZ) - screenZ) <= distThreshZ
%         
            % these are reflections of each other!
            % reflection has a lower z value
            if posMarkers(i, idxZ) > posMarkers(j, idxZ)
                remove(j) = uint8(1);
                foundReflection(i) = uint8(1);
            else
                remove(i) = uint8(1);
                foundReflection(j) = uint8(1);
            end
        end
    end
end

% keep the ones not marked for removal
for i = 1:numMarkers
   if remove(i)
       numReflections = numReflections + uint8(1);
   else
       numMarkersFiltered = numMarkersFiltered + uint8(1);
       posMarkersFiltered(numMarkersFiltered, :) = posMarkers(i,:);
   end
end

end

== matlab function RefModel_RigInput/Serial Quad Card: Polaris, Iscan/Parse Polaris/Filter Volume ==
  data: numMarkers input; numMarkersFiltered output; posMarkers input; rigConfig input; posMarkersFiltered output; numOutOfVolume output
function [numMarkersFiltered, posMarkersFiltered, numOutOfVolume] = filterVolumeApplyOffset(...
    numMarkers, posMarkers, rigConfig)
% distThresh : maximum distance in x,y and from screen for pairs of markers
%   to be considered reflections
% screenZ : the coordinates of the screen plane in Z
% signAwayFromScreen : if 1, the reflection will have a lower Z value than
%   the actual marker, if -1, the reflection will have a higher Z value than
%   the actual marker.

% default values
xLim = rigConfig.polarisVolumeLimsX;
yLim = rigConfig.polarisVolumeLimsY;
zLim = rigConfig.polarisVolumeLimsZ;
origin = rigConfig.polarisOrigin;
offset = rigConfig.polarisManualOffset;

idxX = uint8(1);
idxY = uint8(2);
idxZ = uint8(3);

remove = zeros(size(posMarkers,1), 1, 'uint8');
remove = remove | posMarkers(:, idxX) < xLim(1) | posMarkers(:, idxX) > xLim(2);
remove = remove | posMarkers(:, idxY) < yLim(1) | posMarkers(:, idxY) > yLim(2);
remove = remove | posMarkers(:, idxZ) < zLim(1) | posMarkers(:, idxZ) > zLim(2);

% keep the ones not marked for removal
numOutOfVolume = uint8(0);
posMarkersFiltered = 0*posMarkers;
numMarkersFiltered = uint8(0);
for i = 1:numMarkers
   if remove(i)
       numOutOfVolume = numOutOfVolume + uint8(1);
   else
       numMarkersFiltered = numMarkersFiltered + uint8(1);
       posMarkersFiltered(numMarkersFiltered, :) = posMarkers(i,:) - origin' + offset';
   end
end

end

== matlab function RefModel_RigInput/Serial Quad Card: Polaris, Iscan/Parse Polaris/Extract Marker Position ==
  data: u input uint8; sync output; numMarkersOut output; posMarkersOut output int32; error output; count input
function [sync, numMarkersOut, posMarkersOut, error] = parsePolaris(u, count)

%%%%%%%%%%%%%%%%%%%%%
%
% ShenoyLab
% Paul Nuyujukian
% 3/2009
% 
% Modified by Dan O'Shea djoshea@stanford.edu
% To output multiple Polaris markers
% and to remove the absurdly high counts of magic numbers and undocumented
% offsets littered throughout :)
%
% determine hand position from ascii polaris vector
% for some reason, ascii decode breaks the FIFO read buffer
%     so used embedded matlab function instead
% 
% input vector is a uint8 [1 1025] (FIFO Buffer)
% 21 characters are important, in indexes u(9 29)
% in format of +/-XXXXXX  +/-XXXXXX  +/-XXXXXX
% where:           Tx          Ty        Tz
% and where these are ascii representations of polaris coordinates
% note, there is an implied decimal point for each value: +/-XXXX.XX (in meters)
% decimal point is ignored to keep everything as integer computation
%
%
% numMarkersOut is the number of markers found
% posMarkersOut(i,:) is the [X Y Z] position of marker i
%   it will always have the same number of rows (nMarkersOut defined below)
%   but only the first numMarkersOut rows will contain valid data
% sync is 0 unless a new value has been read, then it goes to 1
%
%%%%%%%%%%%%%%%%%%%%%%%%%%%%%%%%%%%%%%%%

% persistent vars kept across ticks of simulink time
% so that we can keep outputting positions in between hearing from Polaris
persistent numMarkers;
persistent posMarkers;
persistent frameNum;

% defines buffer size
nMarkersBuffer = uint8(10);
CHAR_LF = uint8(10);
CHAR_ZERO = uint8(48);
CHAR_ONE = uint8(49);
CHAR_NINE = uint8(57);
CHAR_A = uint8(65);
CHAR_F = uint8(70);
CHAR_PLUS = uint8(43);
CHAR_MINUS = uint8(45);

ERROR_HEADER = uint8(1);
ERROR_NUMMARKERS_DIGIT1 = uint8(2);
ERROR_NUMMARKERS_DIGIT2 = uint8(3);

% coord errors are ## where the tens place is the marker, the ones is the coordinate
ERROR_COORDSIGN = zeros(nMarkersBuffer, 3, 'uint8');
for i = uint8(1):nMarkersBuffer
    ERROR_COORDSIGN(i, :) = uint8(10*i) + uint8([1 2 3]);
end

emptyPosMarkers = zeros(nMarkersBuffer, 3, 'int32');

% initialize persistents
if(isempty(numMarkers))
    numMarkers = uint8(0);
    posMarkers = zeros(nMarkersBuffer, 3, 'int32');
    frameNum = int32(0);
end

% initialize outputs to equal persistents so that if an error occurs we can
% just return immediately
sync = uint8(0);
numMarkersOut = numMarkers;
posMarkersOut = posMarkers;
frameNumOut = frameNum;
error = uint8(0);

% treat as uint8
in = uint8(u);

if count == 0 || in(1) == uint8(0)
    % no new data, just hold everything till next update
    return;
end

% clear the output buffer so it goes to zero if we hit an error
posMarkers = emptyPosMarkers;

% position in the input buffer to look at
% header has length 5: '0101\n' or '\0101\n' (not sure why the first byte
% is zero, just empirically seems to be so on rig 5)
header = [CHAR_ZERO CHAR_ONE CHAR_ZERO CHAR_ONE CHAR_LF]';

% indicate that we've received a signal and ask Polaris for more
sync = uint8(1);

% check response header
if ~all(in(1:5) == header)
    % just output the values from last time
    error = ERROR_HEADER;
    return;
end
offset = uint8(length(header)+1);

% decode the number of markers
digit1 = in(offset);
digit2 = in(offset+1);
offset = offset + 2;

% decode hex digit 1
if(digit1 >= CHAR_ZERO && digit1 <= CHAR_NINE)
    hex1 = digit1 - CHAR_ZERO;
elseif(digit1 >= CHAR_A && digit1 <= CHAR_F)
    hex1 = digit1 - CHAR_A + 10;
else
    % error!
    hex1 = uint8(0);
    error = ERROR_NUMMARKERS_DIGIT1;
    posMarkers = emptyPosMarkers;
    return;
end

% decode hex digit 2
if(digit2 >= CHAR_ZERO && digit2 <= CHAR_NINE)
    hex2 = digit2 - CHAR_ZERO;
elseif(digit2 >= CHAR_A && digit2 <= CHAR_F)
    hex2 = digit2 - CHAR_A + 10;
else
    hex2 = uint8(0);
    % error!
    error = ERROR_NUMMARKERS_DIGIT2;
    posMarkers = emptyPosMarkers;
    return;
end

% combine 2 digit hex number of markers
numMarkers = hex1*uint8(16) + hex2;

% next is 1 hex character for every 4 markers which is an out of volume
% flag, which we simply skip
offset = offset + uint8(ceil(double(numMarkers) / 4.0));
val = int32(0);
sign = int32(0);

% can only look at first N markers
if numMarkers > nMarkersBuffer
    numMarkers = nMarkersBuffer;
end

% loop over markers, extracting positions
for iMarker = 1:numMarkers

    % loop over x,y,z
    for iCoord = uint8(1:3)
        if in(offset) == CHAR_PLUS
            sign = int32(1);
        elseif in(offset) == CHAR_MINUS
            sign = int32(-1);
        else
            sign = int32(0);
            error = ERROR_COORDSIGN(iMarker, iCoord);
            posMarkers = emptyPosMarkers;
            return;
        end
        offset = offset + 1;

        % decode 6 decimal places per coordinate, and multiply by the sign
        val = sign * sum(int32(int32(in(offset + uint8(1:6)) - CHAR_ZERO).*int32([100000 10000 1000 100 10 1]')));

        offset = offset + 6;
        % store in posMarkers
        posMarkers(iMarker, iCoord) = val;
    end
end

% increment frameNum
frameNum = frameNum + 1;
    
% update with the new values
numMarkersOut = numMarkers;
posMarkersOut = posMarkers;
frameNumOut = frameNum;


end

== matlab function RefModel_RigInput/Serial Quad Card: Polaris, Iscan/Parse Polaris/Request Marker ==
  data: S input uint8; A output uint8 size=9
function A = request_marker(S)
% ascii encode of marker request to polaris
% sent as null terminated string
%
% ascii 13 = carriage return

if (S == 1)
    A = [ uint8('TX 1800') 13 ]'; % command to request marker data
else
    A = zeros(0, 1, 'uint8'); % send nothing
end

== matlab function RefModel_RigInput/Serial Quad Card: Polaris, Iscan/Parse Polaris/Transpose Coordinates ==
  data: u input; out output
function out = convertCoordinates(u)

% Rig X Y Z corresponds to Polaris X Z Y
% Polaris is in 10-micron units = 0.01, Rig is in mm
out = [ double(u(:, 2))/1000.0 double(u(:, 3))/1000.0 double(u(:, 1))/1000.0 ];

== matlab function RefModel_RigInput/Serial Quad Card: Polaris, Iscan/Parse Polaris/kick Polaris ==
  data: sync input; trig output
function trig = kickPolaris(sync)


persistent count;

if isempty(count)
    count = uint16(0);
end

if sync == uint8(1)
    count = uint16(0);
else
    count = count + uint16(1);
end

if count == uint16(1000)
    trig = uint8(1);
    count = uint16(0);
else
    trig = uint8(0);
end

== matlab function RefModel_RigInput/Receive MicroscopeState/Convert Fixed to Variable ==
  data: in input; out output size=bufferSize; N input size=1; bufferSize parameter size=1
function out = fixedToVariable(in, N, bufferSize)
%#codegen

if N == 0
    out = zeros(0, 1, class(in)); %#ok<ZEROLIKE>
elseif N > bufferSize
    out = in;
else
    out = in(1:N);
end

== matlab function RefModel_RigInput/Eye Bus Placeholder ==
  data: bus output Bus: EyeInputBus size=1
function bus = initialize_EyeInputBus()
%#codegen 

    bus = initializeBus_EyeInputBus();

end

== matlab function RefModel_RigInput/Network from Display/Enable after N ms/MATLAB Function3 ==
  data: i1 input uint8; o output uint8 size=1; i2 input uint8 size=1
function o = OR(i1, i2)
%#codegen

o = uint8(i1 || i2);

== matlab function RefModel_RigInput/Network from Display/Logical And ==
  data: i1 input uint8; o output uint8 size=1; i2 input uint8 size=1; i3 input uint8 size=1
function o = AND(i1, i2, i3)
%#codegen

o = uint8(i1 && i2 && i3);

== matlab function RefModel_RigInput/Tunable Rig Config/Deserialize Bus Parameter ==
  data: valAsDouble input double; bus output Bus: RigConfigBus size=1; update output uint8 size=1; allowPending input uint8 size=1; receivedInvalid output uint8 size=1
function [bus, update, receivedInvalid] = deserializeBusParameter(valAsDouble, allowPending)
%#codegen

    % typecast to bytes
    valAsBytes = typecast(valAsDouble, 'uint8');

    % use the first byte as updateCounter, check for whether counter has been incremented
    thisCounter = valAsBytes(1);
    persistent pLastCounter;
    if isempty(pLastCounter)
        pLastCounter = thisCounter;
    end
    if pLastCounter ~= thisCounter
        recvUpdate = uint8(1);
        pLastCounter = thisCounter;
    else
        recvUpdate = uint8(0);
    end
    startOffset = 2;

    % external cached output for when allowPending 
    persistent pBusOut;
    if isempty(pBusOut)
        pBusOut = initializeBus_RigConfigBus();
    end

    % parse incoming bytes if allowing updates
    receivedInvalid = uint8(0);
    if allowPending
        [bus, valid] = deserializeBus_RigConfigBus(valAsBytes, startOffset);
        if valid
            % update internal cache
            pBusOut = bus;
        else
            % don't update internal cache, output internal cache
            bus = pBusOut;
            receivedInvalid = uint8(1);
            recvUpdate = uint8(0);
        end
    else
        bus = pBusOut;
    end

    % track whether we have a pending update
    persistent pPending;
    if isempty(pPending), pPending = uint8(0); end
    if recvUpdate
        if allowPending
            % update goes out immediately
            update = uint8(1);
            pPending = uint8(0);
        else
            % queue pending update
            update = uint8(0);
            pPending = uint8(1);
        end
    else
        if allowPending
            % release pending
            update = pPending;
            pPending = uint8(0);
        else
            % do nothing
            update = uint8(0);
        end
    end

    % reset fields marked with .resetImmediately immediately after update
    if ~update

    end
end
